simulink model "Stage_4_CAN_Fault_Diagnostics"  (R2025a)
settings: Solver=VariableStepAuto  StartTime=0.0  StopTime=10  RelTol=1e-3
libraries: SignalEditorBlockLib x12, canmsglib x8, simulink x1
settings Model: Creator=sitam  LastModifiedBy=sitam

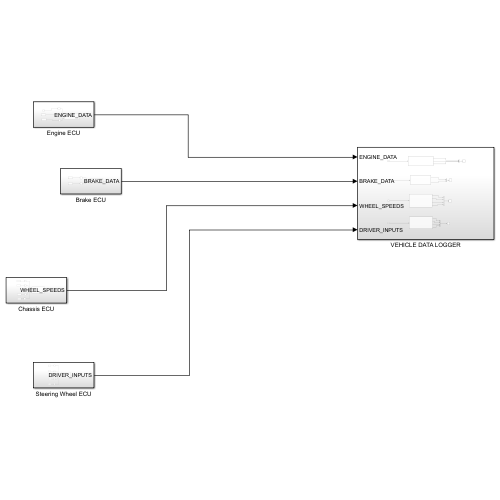
[thumbnail: Simulink's stored preview of the top-level diagram]
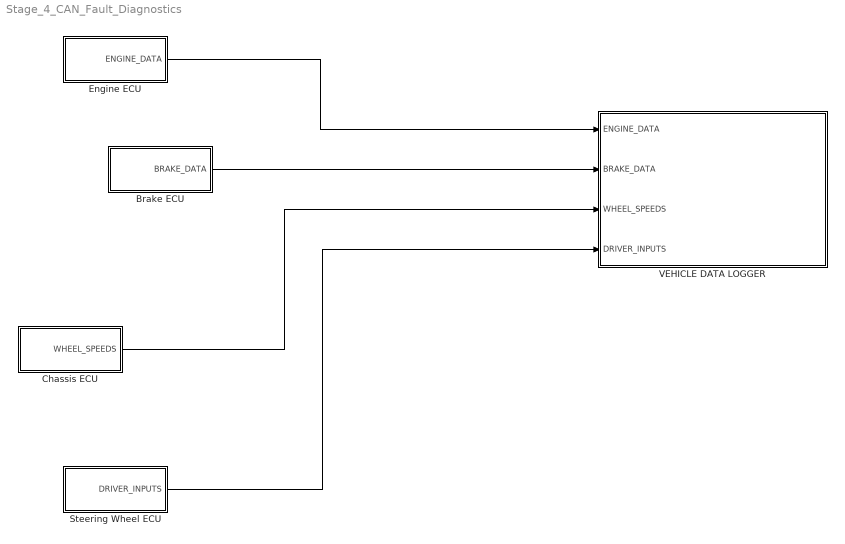
== system Stage_4_CAN_Fault_Diagnostics ==
  Brake ECU : Subsystem
  Chassis ECU : Subsystem
  Engine ECU : Subsystem
  Steering Wheel ECU : Subsystem
  VEHICLE DATA LOGGER : Subsystem
  wires:
  Engine ECU/1(ENGINE_DATA) -> VEHICLE DATA LOGGER/1(ENGINE_DATA)
  Brake ECU/1(BRAKE_DATA) -> VEHICLE DATA LOGGER/2(BRAKE_DATA)
  Chassis ECU/1(WHEEL_SPEEDS) -> VEHICLE DATA LOGGER/3(WHEEL_SPEEDS)
  Steering Wheel ECU/1(DRIVER_INPUTS) -> VEHICLE DATA LOGGER/4(DRIVER_INPUTS)

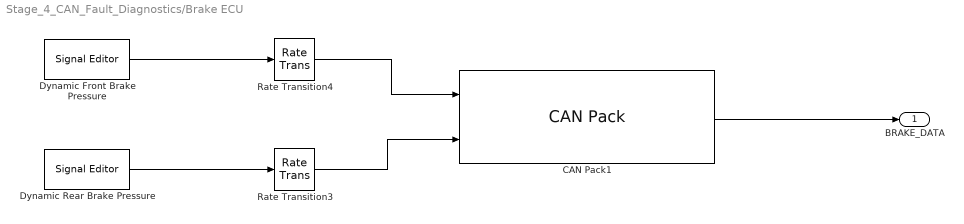
== system Stage_4_CAN_Fault_Diagnostics/Brake ECU ==
  CAN Pack1 : canmsglib/CAN Pack  CANdbFile=C:\Users\sitam\OneDrive\Projects\CAN Bus Project\MotorsportCAN.dbc  MsgList=BRAKE_DATA  MsgName=BRAKE_DATA  MsgIDType=Standard (11-bit identifier)  MsgIdentifier=512  CANIDInput=off  MsgLength=8  Remote=off  ApplyMinMax=off  BusOutput=off  SignalInfo={'FrontBrakePressure','0','16','LE','unsigned','Standard','0','0.01','0','0','200';'RearBrakePressure','16','16','LE','unsigned','Standard','0','0.01','0','0','200'}
      settings: LibrarySourceBlock=canlib/CAN Pack  DataFormat=CANdb specified signals
  Dynamic Front Brake Pressure : SignalEditorBlockLib/Signal Editor  FileName=3_frontbrake.mat  ActiveScenario=Scenario  ActiveSignal=Signal 1  IsBus=off  OutputBusObjectStr=Bus: BusObject  SampleTime=0  ZeroCross=off  OutputAfterFinalValue=Setting to zero  Unit=inherit  PreserveSignalName=on  ApplySigPropsToAllScenarios=on  ApplySigPropsToAllSignals=off  SignalPropertySource=Dialog parameters
  Dynamic Rear Brake Pressure : SignalEditorBlockLib/Signal Editor  FileName=3_rearbrake.mat  ActiveScenario=Scenario  ActiveSignal=Signal 1  IsBus=off  OutputBusObjectStr=Bus: BusObject  SampleTime=0  ZeroCross=off  OutputAfterFinalValue=Setting to zero  Unit=inherit  PreserveSignalName=on  ApplySigPropsToAllScenarios=on  ApplySigPropsToAllSignals=off  SignalPropertySource=Dialog parameters
  Rate Transition3 : RateTransition  OutPortSampleTime=0.01
  Rate Transition4 : RateTransition  OutPortSampleTime=0.01
  BRAKE_DATA : Outport
  wires:
  Rate Transition4/1 -> CAN Pack1/1
  Rate Transition3/1 -> CAN Pack1/2
  CAN Pack1/1 -> BRAKE_DATA/1
  Dynamic Front Brake Pressure/1 -> Rate Transition4/1
  Dynamic Rear Brake Pressure/1 -> Rate Transition3/1

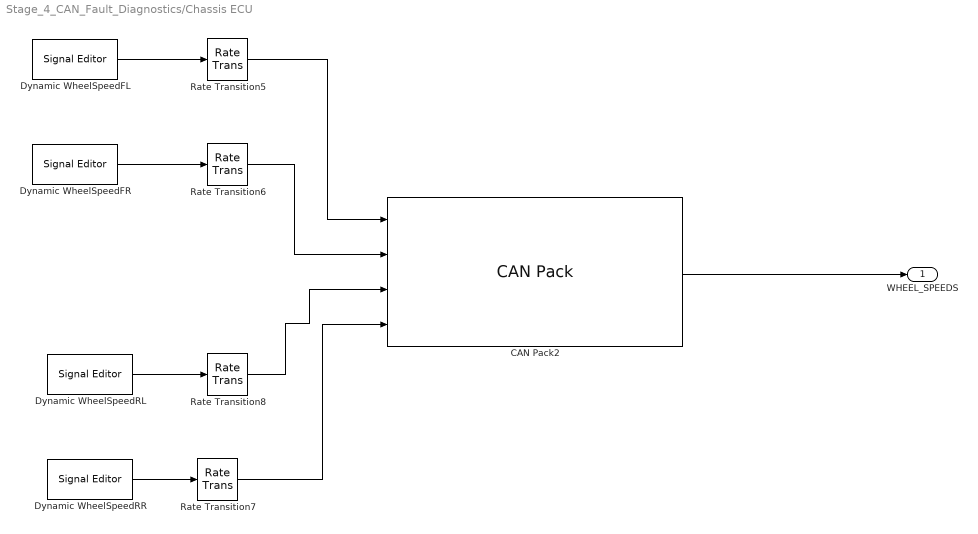
== system Stage_4_CAN_Fault_Diagnostics/Chassis ECU ==
  CAN Pack2 : canmsglib/CAN Pack  CANdbFile=C:\Users\sitam\OneDrive\Projects\CAN Bus Project\MotorsportCAN.dbc  MsgList=WHEEL_SPEEDS  MsgName=WHEEL_SPEEDS  MsgIDType=Standard (11-bit identifier)  MsgIdentifier=768  CANIDInput=off  MsgLength=8  Remote=off  ApplyMinMax=off  BusOutput=off  SignalInfo={'WheelSpeedFL','0','16','LE','unsigned','Standard','0','0.01','0','0','350';'WheelSpeedFR','16','16','LE','unsigned','Standard','0','0.01','0','0','350';'WheelSpeedRL','32','16','LE','unsigned','Standard','0','0.01','0','0','350';'WheelSpeedRR','48','16','LE','unsigned','Standard','0','0.01','0','0','350'}
      settings: LibrarySourceBlock=canlib/CAN Pack  DataFormat=CANdb specified signals
  Dynamic WheelSpeedFL : SignalEditorBlockLib/Signal Editor  FileName=3_WheelSpeedFL.mat  ActiveScenario=Scenario  ActiveSignal=Signal 1  IsBus=off  OutputBusObjectStr=Bus: BusObject  SampleTime=0  ZeroCross=off  OutputAfterFinalValue=Setting to zero  Unit=inherit  PreserveSignalName=on  ApplySigPropsToAllScenarios=on  ApplySigPropsToAllSignals=off  SignalPropertySource=Dialog parameters
  Dynamic WheelSpeedFR : SignalEditorBlockLib/Signal Editor  FileName=3_WheelSpeedFR.mat  ActiveScenario=Scenario  ActiveSignal=Signal 1  IsBus=off  OutputBusObjectStr=Bus: BusObject  SampleTime=0  ZeroCross=off  OutputAfterFinalValue=Setting to zero  Unit=inherit  PreserveSignalName=on  ApplySigPropsToAllScenarios=on  ApplySigPropsToAllSignals=off  SignalPropertySource=Dialog parameters
  Dynamic WheelSpeedRL : SignalEditorBlockLib/Signal Editor  FileName=3_WheelSpeedRL.mat  ActiveScenario=Scenario  ActiveSignal=Signal 1  IsBus=off  OutputBusObjectStr=Bus: BusObject  SampleTime=0  ZeroCross=off  OutputAfterFinalValue=Setting to zero  Unit=inherit  PreserveSignalName=on  ApplySigPropsToAllScenarios=on  ApplySigPropsToAllSignals=off  SignalPropertySource=Dialog parameters
  Dynamic WheelSpeedRR : SignalEditorBlockLib/Signal Editor  FileName=3_WheelSpeedRR.mat  ActiveScenario=Scenario  ActiveSignal=Signal 1  IsBus=off  OutputBusObjectStr=Bus: BusObject  SampleTime=0  ZeroCross=off  OutputAfterFinalValue=Setting to zero  Unit=inherit  PreserveSignalName=on  ApplySigPropsToAllScenarios=on  ApplySigPropsToAllSignals=off  SignalPropertySource=Dialog parameters
  Rate Transition{5..8} (4 alike) : RateTransition  OutPortSampleTime=0.005
  WHEEL_SPEEDS : Outport
  wires:
  Rate Transition8/1 -> CAN Pack2/3
  CAN Pack2/1 -> WHEEL_SPEEDS/1
  Dynamic WheelSpeedFL/1 -> Rate Transition5/1
  Dynamic WheelSpeedFR/1 -> Rate Transition6/1
  Dynamic WheelSpeedRL/1 -> Rate Transition8/1
  Rate Transition5/1 -> CAN Pack2/1
  Dynamic WheelSpeedRR/1 -> Rate Transition7/1
  Rate Transition7/1 -> CAN Pack2/4
  Rate Transition6/1 -> CAN Pack2/2

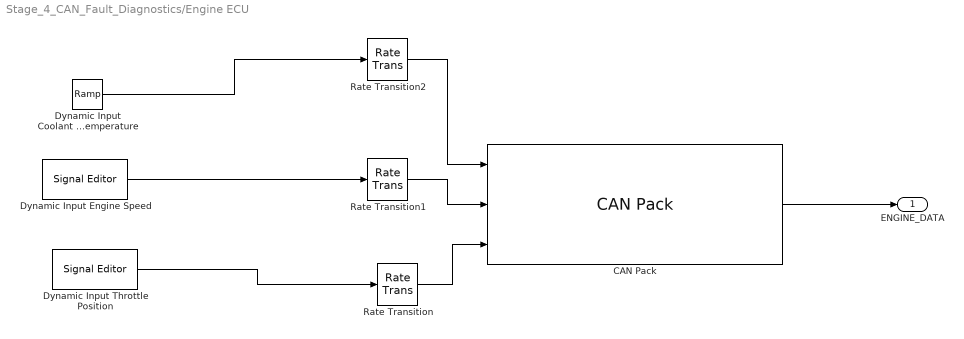
== system Stage_4_CAN_Fault_Diagnostics/Engine ECU ==
  CAN Pack : canmsglib/CAN Pack  CANdbFile=C:\Users\sitam\OneDrive\Projects\CAN Bus Project\MotorsportCAN.dbc  MsgList=ENGINE_DATA  MsgName=ENGINE_DATA  MsgIDType=Standard (11-bit identifier)  MsgIdentifier=256  CANIDInput=off  MsgLength=8  Remote=off  ApplyMinMax=off  BusOutput=off  SignalInfo={'CoolantTemperature','24','8','LE','unsigned','Standard','0','1','-40','-40','150';'EngineSpeed','0','16','LE','unsigned','Standard','0','0.25','0','0','15000';'ThrottlePosition','16','8','LE','unsigned','Standard','0','0.4','0','0','100'}
      settings: LibrarySourceBlock=canlib/CAN Pack  DataFormat=CANdb specified signals
  Dynamic Input Coolant Temperature : simulink/Sources/Ramp  slope=1  start=0  InitialOutput=85
  Dynamic Input Engine Speed : SignalEditorBlockLib/Signal Editor  FileName=2_2-enginespeed.mat  ActiveScenario=Scenario  ActiveSignal=Signal 1  IsBus=off  OutputBusObjectStr=Bus: BusObject  SampleTime=0  ZeroCross=off  OutputAfterFinalValue=Setting to zero  Unit=inherit  PreserveSignalName=on  ApplySigPropsToAllScenarios=on  ApplySigPropsToAllSignals=off  SignalPropertySource=Dialog parameters
  Dynamic Input Throttle Position : SignalEditorBlockLib/Signal Editor  FileName=2_2-throttlepos.mat  ActiveScenario=Scenario  ActiveSignal=Signal 1  IsBus=off  OutputBusObjectStr=Bus: BusObject  SampleTime=0  ZeroCross=off  OutputAfterFinalValue=Setting to zero  Unit=inherit  PreserveSignalName=on  ApplySigPropsToAllScenarios=on  ApplySigPropsToAllSignals=off  SignalPropertySource=Dialog parameters
  Rate Transition : RateTransition  OutPortSampleTime=0.01
  Rate Transition1 : RateTransition  OutPortSampleTime=0.01
  Rate Transition2 : RateTransition  OutPortSampleTime=0.01
  ENGINE_DATA : Outport
  wires:
  CAN Pack/1 -> ENGINE_DATA/1
  Dynamic Input Coolant Temperature/1 -> Rate Transition2/1
  Rate Transition2/1 -> CAN Pack/1
  Dynamic Input Engine Speed/1 -> Rate Transition1/1
  Rate Transition1/1 -> CAN Pack/2
  Dynamic Input Throttle Position/1 -> Rate Transition/1
  Rate Transition/1 -> CAN Pack/3

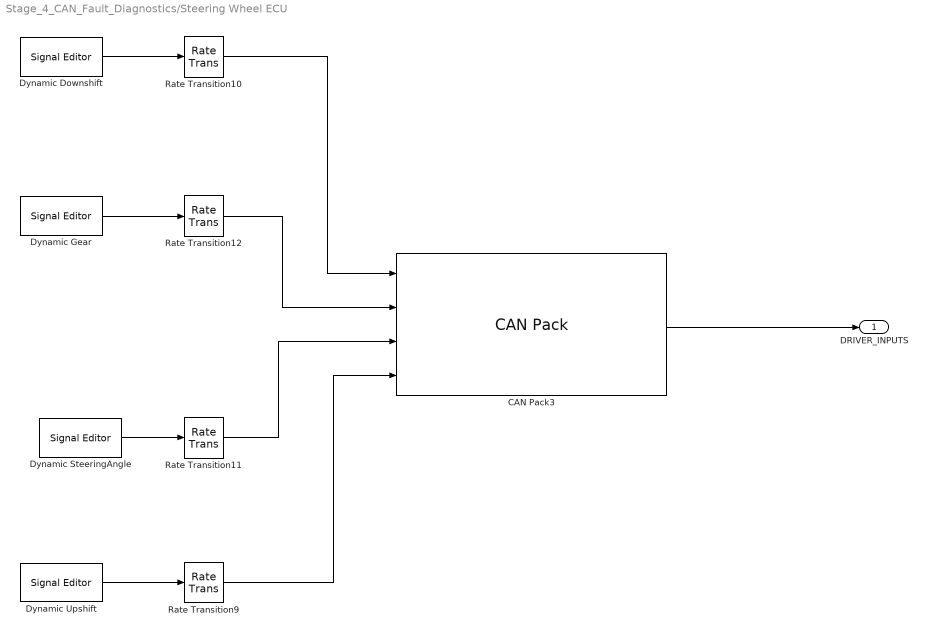
== system Stage_4_CAN_Fault_Diagnostics/Steering Wheel ECU ==
  CAN Pack3 : canmsglib/CAN Pack  CANdbFile=C:\Users\sitam\OneDrive\Projects\CAN Bus Project\MotorsportCAN.dbc  MsgList=DRIVER_INPUTS  MsgName=DRIVER_INPUTS  MsgIDType=Standard (11-bit identifier)  MsgIdentifier=1024  CANIDInput=off  MsgLength=8  Remote=off  ApplyMinMax=off  BusOutput=off  SignalInfo={'Downshift','25','1','LE','unsigned','Standard','0','1','0','0','1';'Gear','16','3','LE','unsigned','Standard','0','1','0','0','7';'SteeringAngle','0','16','LE','signed','Standard','0','0.1','0','-540','540';'Upshift','24','1','LE','unsigned','Standard','0','1','0','0','1'}
      settings: LibrarySourceBlock=canlib/CAN Pack  DataFormat=CANdb specified signals
  Dynamic Downshift : SignalEditorBlockLib/Signal Editor  FileName=3_downshift.mat  ActiveScenario=Scenario  ActiveSignal=Signal 1  IsBus=off  OutputBusObjectStr=Bus: BusObject  SampleTime=0  ZeroCross=off  OutputAfterFinalValue=Setting to zero  Unit=inherit  PreserveSignalName=on  ApplySigPropsToAllScenarios=on  ApplySigPropsToAllSignals=off  SignalPropertySource=Dialog parameters
  Dynamic Gear : SignalEditorBlockLib/Signal Editor  FileName=3_gear.mat  ActiveScenario=Scenario  ActiveSignal=Signal 1  IsBus=off  OutputBusObjectStr=Bus: BusObject  SampleTime=0  ZeroCross=off  OutputAfterFinalValue=Setting to zero  Unit=inherit  PreserveSignalName=on  ApplySigPropsToAllScenarios=on  ApplySigPropsToAllSignals=off  SignalPropertySource=Dialog parameters
  Dynamic SteeringAngle : SignalEditorBlockLib/Signal Editor  FileName=3_steeringangle.mat  ActiveScenario=Scenario  ActiveSignal=Signal 1  IsBus=off  OutputBusObjectStr=Bus: BusObject  SampleTime=0  ZeroCross=off  OutputAfterFinalValue=Setting to zero  Unit=inherit  PreserveSignalName=on  ApplySigPropsToAllScenarios=on  ApplySigPropsToAllSignals=off  SignalPropertySource=Dialog parameters
  Dynamic Upshift : SignalEditorBlockLib/Signal Editor  FileName=3_upshift.mat  ActiveScenario=Scenario  ActiveSignal=Signal 1  IsBus=off  OutputBusObjectStr=Bus: BusObject  SampleTime=0  ZeroCross=off  OutputAfterFinalValue=Setting to zero  Unit=inherit  PreserveSignalName=on  ApplySigPropsToAllScenarios=on  ApplySigPropsToAllSignals=off  SignalPropertySource=Dialog parameters
  Rate Transition{9..12} (4 alike) : RateTransition  OutPortSampleTime=0.02
  DRIVER_INPUTS : Outport
  wires:
  Rate Transition10/1 -> CAN Pack3/1
  Dynamic Upshift/1 -> Rate Transition9/1
  Rate Transition11/1 -> CAN Pack3/3
  Dynamic SteeringAngle/1 -> Rate Transition11/1
  Rate Transition9/1 -> CAN Pack3/4
  Rate Transition12/1 -> CAN Pack3/2
  Dynamic Gear/1 -> Rate Transition12/1
  Dynamic Downshift/1 -> Rate Transition10/1
  CAN Pack3/1 -> DRIVER_INPUTS/1

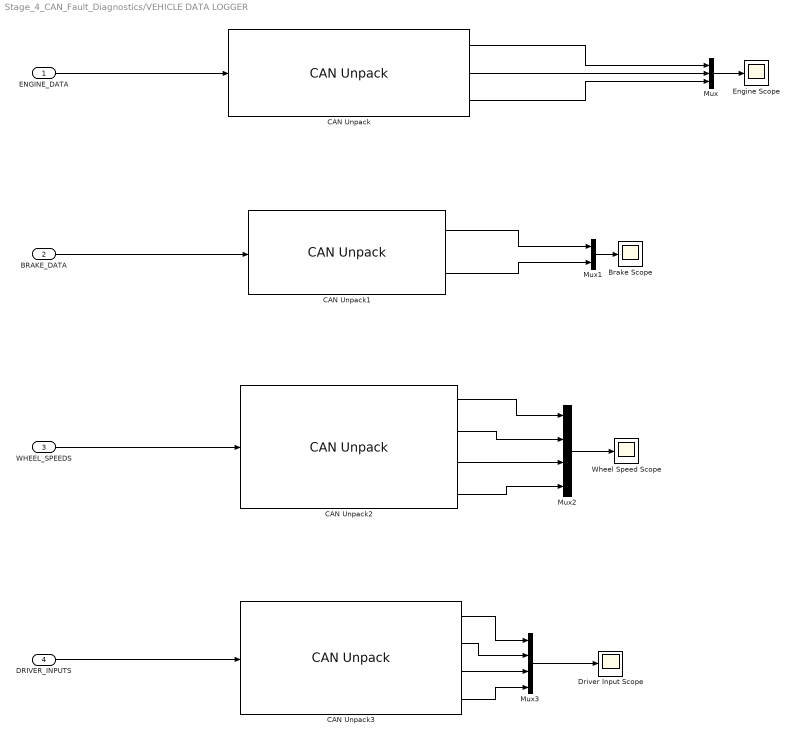
== system Stage_4_CAN_Fault_Diagnostics/VEHICLE DATA LOGGER ==
  ENGINE_DATA : Inport
  BRAKE_DATA : Inport  Port=2
  WHEEL_SPEEDS : Inport  Port=3
  DRIVER_INPUTS : Inport  Port=4
  Brake Scope : Scope
      settings: ActiveDisplayYMinimum=-14.999999999999996  ActiveDisplayYMaximum=135  DataLoggingVariableName=ScopeData15
  CAN Unpack : canmsglib/CAN Unpack  CANdbFile=C:\Users\sitam\OneDrive\Projects\CAN Bus Project\MotorsportCAN.dbc  MsgList=ENGINE_DATA  MsgName=ENGINE_DATA  MsgIDType=Standard (11-bit identifier)  MsgIdentifier=256  MsgLength=8  SignalInfo={'CoolantTemperature','24','8','LE','unsigned','Standard','0','1','-40','-40','150';'EngineSpeed','0','16','LE','unsigned','Standard','0','0.25','0','0','15000';'ThrottlePosition','16','8','LE','unsigned','Standard','0','0.4','0','0','100'}  IDPort=off  TimestampPort=off  ErrorPort=off  RemotePort=off  LengthPort=off  StatusPort=off  ApplyMinMax=off
      settings: LibrarySourceBlock=canlib/CAN Unpack  DataFormat=CANdb specified signals
  CAN Unpack1 : canmsglib/CAN Unpack  CANdbFile=C:\Users\sitam\OneDrive\Projects\CAN Bus Project\MotorsportCAN.dbc  MsgList=BRAKE_DATA  MsgName=BRAKE_DATA  MsgIDType=Standard (11-bit identifier)  MsgIdentifier=512  MsgLength=8  SignalInfo={'FrontBrakePressure','0','16','LE','unsigned','Standard','0','0.01','0','0','200';'RearBrakePressure','16','16','LE','unsigned','Standard','0','0.01','0','0','200'}  IDPort=off  TimestampPort=off  ErrorPort=off  RemotePort=off  LengthPort=off  StatusPort=off  ApplyMinMax=off
      settings: LibrarySourceBlock=canlib/CAN Unpack  DataFormat=CANdb specified signals
  CAN Unpack2 : canmsglib/CAN Unpack  CANdbFile=C:\Users\sitam\OneDrive\Projects\CAN Bus Project\MotorsportCAN.dbc  MsgList=WHEEL_SPEEDS  MsgName=WHEEL_SPEEDS  MsgIDType=Standard (11-bit identifier)  MsgIdentifier=768  MsgLength=8  SignalInfo={'WheelSpeedFL','0','16','LE','unsigned','Standard','0','0.01','0','0','350';'WheelSpeedFR','16','16','LE','unsigned','Standard','0','0.01','0','0','350';'WheelSpeedRL','32','16','LE','unsigned','Standard','0','0.01','0','0','350';'WheelSpeedRR','48','16','LE','unsigned','Standard','0','0.01','0','0','350'}  IDPort=off  TimestampPort=off  ErrorPort=off  RemotePort=off  LengthPort=off  StatusPort=off  ApplyMinMax=off
      settings: LibrarySourceBlock=canlib/CAN Unpack  DataFormat=CANdb specified signals
  CAN Unpack3 : canmsglib/CAN Unpack  CANdbFile=C:\Users\sitam\OneDrive\Projects\CAN Bus Project\MotorsportCAN.dbc  MsgList=DRIVER_INPUTS  MsgName=DRIVER_INPUTS  MsgIDType=Standard (11-bit identifier)  MsgIdentifier=1024  MsgLength=8  SignalInfo={'Downshift','25','1','LE','unsigned','Standard','0','1','0','0','1';'Gear','16','3','LE','unsigned','Standard','0','1','0','0','7';'SteeringAngle','0','16','LE','signed','Standard','0','0.1','0','-540','540';'Upshift','24','1','LE','unsigned','Standard','0','1','0','0','1'}  IDPort=off  TimestampPort=off  ErrorPort=off  RemotePort=off  LengthPort=off  StatusPort=off  ApplyMinMax=off
      settings: LibrarySourceBlock=canlib/CAN Unpack  DataFormat=CANdb specified signals
  Driver Input Scope : Scope
      settings: ActiveDisplayYMinimum=-149.00944352064721  ActiveDisplayYMaximum=158.80440759196159  DataLoggingVariableName=ScopeData13
  Engine Scope : Scope
      settings: ActiveDisplayYMinimum=-910.846129077574  ActiveDisplayYMaximum=12046.717848894572  DataLoggingVariableName=ScopeData16
  Mux : Mux  Inputs=3
  Mux1 : Mux  Inputs=2
  Mux2 : Mux
  Mux3 : Mux
  Wheel Speed Scope : Scope
      settings: ActiveDisplayYMinimum=33.586083369518022  ActiveDisplayYMaximum=140.72894051237517  DataLoggingVariableName=ScopeData14
  wires:
  ENGINE_DATA/1 -> CAN Unpack/1
  DRIVER_INPUTS/1 -> CAN Unpack3/1
  WHEEL_SPEEDS/1 -> CAN Unpack2/1
  BRAKE_DATA/1 -> CAN Unpack1/1
  CAN Unpack/1 -> Mux/1
  CAN Unpack/2 -> Mux/2
  CAN Unpack/3 -> Mux/3
  CAN Unpack1/1 -> Mux1/1
  CAN Unpack1/2 -> Mux1/2
  CAN Unpack2/1 -> Mux2/1
  CAN Unpack2/2 -> Mux2/2
  CAN Unpack2/3 -> Mux2/3
  CAN Unpack2/4 -> Mux2/4
  CAN Unpack3/1 -> Mux3/1
  CAN Unpack3/2 -> Mux3/2
  CAN Unpack3/3 -> Mux3/3
  CAN Unpack3/4 -> Mux3/4
  Mux3/1 -> Driver Input Scope/1
  Mux2/1 -> Wheel Speed Scope/1
  Mux1/1 -> Brake Scope/1
  Mux/1 -> Engine Scope/1
